simulink model "HSat_orbit_merged_maria"  (R2023b)
settings: Solver=FixedStepAuto  StartTime=0  StopTime=86400*900  MaxStep=3600  RelTol=1e-3  EnableMultiTasking=on
values from neighbouring files (symbols this model uses):
  alpha_acc = sqrt(0.7)    [HSat_op_setup_merged_maria.m]    (also in init_orbit_analysis_with_drag_loss.m)
  ext_ENV_G = 6.674e-11    [HSat_op_setup.m]    (also in HSat_op_setup_merged_maria.m)
  ext_ENV_muEarth = 3.986005e14    (= 398600500000000)    [GEO_insertion_setup.m]    (also in HSat_op_setup.m; HSat_op_setup_merged_maria.m; init_orbit_analysis_with_drag_loss.m)
  ext_ENV_Re = 6.37813700*10^6    (= 6378137)    [HSat_op_setup.m]    (also in HSat_op_setup_merged_maria.m)
  ext_EOR_atmosphere_end = 1000e3    (= 1000000)    [HSat_op_setup.m]    (also in HSat_op_setup_merged_maria.m)
  ext_EOR_perigeeraise_end = 600e3    (= 600000)    [HSat_op_setup.m]    (also in HSat_op_setup_merged_maria.m)
  ext_Main_initDate_IC_T = sim_start    [HSat_op_setup.m]    (also in HSat_op_setup_merged_maria.m)
  ext_SC_activecorr_COE_ECI = [1, 1, 1, 0, 0, 0, 0, 0 ]    [HSat_op_setup.m]    (also in HSat_op_setup_merged_maria.m)
  ext_SC_balanced_COE_ECI = [ .500    0.70    1.100 1 1]    [HSat_op_setup.m]    (also in HSat_op_setup_merged_maria.m = [ 0.10 2.10 1.40    1.0000    1.0000]; launch_settings.m)
  ext_SC_cutofferror_COE_ECI = [150e3, .01, 0.1*pi/180, .1*pi/180,.1*pi/180, 0, 0, 0]    [HSat_op_setup.m]    (also in HSat_op_setup_merged_maria.m)
  ext_SC_init_COE_ECI = [a0,ecc0,i0,an0,ap0,tran0,eccan0,ma0]    [HSat_op_setup.m]    (also in HSat_op_setup_merged_maria.m)
  ext_SC_target_COE_ECI = [a1,ecc1,i1,an1,ap1,tran1,eccan1,ma1]    [HSat_op_setup.m]    (also in HSat_op_setup_merged_maria.m)
  ext_SC_target_lambda = 67*pi/180    (= 1.16937059884)    [HSat_op_setup.m]    (also in HSat_op_setup_merged_maria.m)
  flip_timer = 2*60*60    (= 7200)    [HSat_op_setup_merged_maria.m]
  P_solar = 4.56e-6    (= 4.56e-06)    [HSat_op_setup_merged_maria.m]    (also in init_orbit_analysis_with_drag_loss.m)
  sim_SC_init_CoG_EOR_dry = [-0.00448 0.00106 0.46931]    [HSat_op_setup.m]    (also in HSat_op_setup_merged_maria.m)
  sim_SC_init_CoG_propellant = [0 0 0.24758]    [HSat_op_setup.m]    (also in HSat_op_setup_merged_maria.m)
  sim_SC_init_dry_mass = sim_SC_init_wet_mass-sim_SC_init_propellant_mass    (= 727)    [HSat_op_setup.m]    (also in HSat_op_setup_merged_maria.m = 813.7)
  sim_SC_init_MoI_EOR_wet = [ ... (first row only)    [HSat_op_setup.m]    (also in HSat_op_setup_merged_maria.m; init_orbit_analysis_with_drag_loss.m)
  sim_SC_init_wet_mass = 750    [HSat_op_setup.m]    (also in HSat_op_setup_merged_maria.m)
  sim_thrust_force = [ ... (first row only)    [HSat_op_setup.m]    (also in HSat_op_setup_merged_maria.m)
  sim_thrust_massflow = [ ... (first row only)    [HSat_op_setup.m]    (also in HSat_op_setup_merged_maria.m)
  sim_thrust_vector = [ ... (first row only)    [HSat_op_setup.m]    (also in HSat_op_setup_merged_maria.m)
  sim_thruster_position = [ ... (first row only)    [HSat_op_setup.m]    (also in HSat_op_setup_merged_maria.m)
  sim_ts_save = 60    [HSat_op_setup.m]    (also in HSat_op_setup_merged_maria.m)
  sun_pointing_SA = 0    [HSat_op_setup_merged_maria.m]    (also in init_orbit_analysis_with_drag_loss.m)
  third_body_jupiter = 1    [HSat_op_setup.m]    (also in HSat_op_setup_merged_maria.m)
  third_body_moon = 1    [HSat_op_setup.m]    (also in HSat_op_setup_merged_maria.m)
  third_body_sun = 1    [HSat_op_setup.m]    (also in HSat_op_setup_merged_maria.m)
libraries: aerolibutil x59, simulink x18, matrix_library x16, Toolbox x10, sharedtransform x9, sharedutil x5, aerolibatmos2 x1, simulink_extras x1
(part 7 of 8)

== system HSat_orbit_merged_maria/Subsystem1/control/EORattitude/Subsystem4/Attitude for OR thrusters/q_scb_calc/Yscb x Zscb ==
  a(1) a(2) a(3) : Inport
  b(1) b(2) b(3) : Inport  Port=2
  Product : Product  InputSameDT=on  SaturateOnIntegerOverflow=on  OutDataTypeStr=Inherit: Same as first input
  Product1 : Product  InputSameDT=on  SaturateOnIntegerOverflow=on  OutDataTypeStr=Inherit: Same as first input
  Selector : Selector  InputPortWidth=3  IndexOptions=Index vector (dialog)  Indices=[2 3 1]  OutputSizes=1
  Selector1 : Selector  InputPortWidth=3  IndexOptions=Index vector (dialog)  Indices=[3 1 2]  OutputSizes=1
  Selector2 : Selector  InputPortWidth=3  IndexOptions=Index vector (dialog)  Indices=[2 3 1]  OutputSizes=1
  Selector3 : Selector  InputPortWidth=3  IndexOptions=Index vector (dialog)  Indices=[3 1 2]  OutputSizes=1
  Sum : Sum  Inputs=+|-  InputSameDT=on  SaturateOnIntegerOverflow=on  OutDataTypeStr=Inherit: Same as first input
  c(1) c(2) c(3) : Outport  InitialOutput=0
  wires:
  Sum/1 -> c(1) c(2) c(3)/1
  b(1) b(2) b(3)/1 -> Selector1/1, Selector2/1
  Selector/1 -> Product/1
  a(1) a(2) a(3)/1 -> Selector/1, Selector3/1
  Product/1 -> Sum/1
  Selector1/1 -> Product/2
  Product1/1 -> Sum/2
  Selector2/1 -> Product1/2
  Selector3/1 -> Product1/1

== system HSat_orbit_merged_maria/Subsystem1/control/EORattitude/Subsystem4/Attitude for OR thrusters/q_scb_calc/Zeci x Reci ==
  a(1) a(2) a(3) : Inport
  b(1) b(2) b(3) : Inport  Port=2
  Product : Product  InputSameDT=on  SaturateOnIntegerOverflow=on  OutDataTypeStr=Inherit: Same as first input
  Product1 : Product  InputSameDT=on  SaturateOnIntegerOverflow=on  OutDataTypeStr=Inherit: Same as first input
  Selector : Selector  InputPortWidth=3  IndexOptions=Index vector (dialog)  Indices=[2 3 1]  OutputSizes=1
  Selector1 : Selector  InputPortWidth=3  IndexOptions=Index vector (dialog)  Indices=[3 1 2]  OutputSizes=1
  Selector2 : Selector  InputPortWidth=3  IndexOptions=Index vector (dialog)  Indices=[2 3 1]  OutputSizes=1
  Selector3 : Selector  InputPortWidth=3  IndexOptions=Index vector (dialog)  Indices=[3 1 2]  OutputSizes=1
  Sum : Sum  Inputs=+|-  InputSameDT=on  SaturateOnIntegerOverflow=on  OutDataTypeStr=Inherit: Same as first input
  c(1) c(2) c(3) : Outport  InitialOutput=0
  wires:
  Selector3/1 -> Product1/1
  Selector2/1 -> Product1/2
  Product1/1 -> Sum/2
  Selector1/1 -> Product/2
  Product/1 -> Sum/1
  a(1) a(2) a(3)/1 -> Selector3/1, Selector/1
  Selector/1 -> Product/1
  b(1) b(2) b(3)/1 -> Selector2/1, Selector1/1
  Sum/1 -> c(1) c(2) c(3)/1

== system HSat_orbit_merged_maria/Subsystem1/control/EORattitude/Subsystem4/Attitude for SK unloading/Subsystem/VecNormalize4 ==
  In1 : Inport
  Constant : Constant
  Demux : Demux  Outputs=[-1 1]
  Divide : Product  Inputs=*/  OutDataTypeStr=double
  Ground : Ground
  Math Function : Math  Operator=square  SignedPower=on
  Math Function1 : Math  Operator=sqrt  SignedPower=on
  Mux : Mux  Inputs=2
  Mux1 : Mux  Inputs=2
  Product : Product  RndMeth=Zero
  Sum of Elements : Sum  Inputs=+
  Switch : Switch  Criteria=u2 > Threshold  Threshold=eps  SaturateOnIntegerOverflow=off  InputSameDT=off
  Out1 : Outport  VectorParamsAs1DForOutWhenUnconnected=off
  wires:
  Math Function/1 -> Sum of Elements/1
  Demux/1 -> Divide/1
  Constant/1 -> Mux1/2
  Mux1/1 -> Switch/3
  Divide/1 -> Out1/1
  Switch/1 -> Demux/1
  Mux/1 -> Switch/1
  Demux/2 -> Divide/2
  Product/1 -> Mux1/1
  In1/1 -> Product/1, Math Function/1, Mux/1
  Ground/1 -> Product/2
  Sum of Elements/1 -> Math Function1/1
  Math Function1/1 -> Mux/2, Switch/2

== system HSat_orbit_merged_maria/Subsystem1/control/EORattitude/Subsystem4/Attitude for SK unloading/Subsystem/Zeci x Reci ==
  a(1) a(2) a(3) : Inport
  b(1) b(2) b(3) : Inport  Port=2
  Product : Product  InputSameDT=on  SaturateOnIntegerOverflow=on  OutDataTypeStr=Inherit: Same as first input
  Product1 : Product  InputSameDT=on  SaturateOnIntegerOverflow=on  OutDataTypeStr=Inherit: Same as first input
  Selector : Selector  InputPortWidth=3  IndexOptions=Index vector (dialog)  Indices=[2 3 1]  OutputSizes=1
  Selector1 : Selector  InputPortWidth=3  IndexOptions=Index vector (dialog)  Indices=[3 1 2]  OutputSizes=1
  Selector2 : Selector  InputPortWidth=3  IndexOptions=Index vector (dialog)  Indices=[2 3 1]  OutputSizes=1
  Selector3 : Selector  InputPortWidth=3  IndexOptions=Index vector (dialog)  Indices=[3 1 2]  OutputSizes=1
  Sum : Sum  Inputs=+|-  InputSameDT=on  SaturateOnIntegerOverflow=on  OutDataTypeStr=Inherit: Same as first input
  c(1) c(2) c(3) : Outport  InitialOutput=0
  wires:
  Selector3/1 -> Product1/1
  Selector2/1 -> Product1/2
  Product1/1 -> Sum/2
  Selector1/1 -> Product/2
  Product/1 -> Sum/1
  a(1) a(2) a(3)/1 -> Selector3/1, Selector/1
  Selector/1 -> Product/1
  b(1) b(2) b(3)/1 -> Selector2/1, Selector1/1
  Sum/1 -> c(1) c(2) c(3)/1

== system HSat_orbit_merged_maria/Subsystem1/control/EORattitude/Subsystem4/Attitude for SK unloading/Subsystem/Zeci x Reci1 ==
  a(1) a(2) a(3) : Inport
  b(1) b(2) b(3) : Inport  Port=2
  Product : Product  InputSameDT=on  SaturateOnIntegerOverflow=on  OutDataTypeStr=Inherit: Same as first input
  Product1 : Product  InputSameDT=on  SaturateOnIntegerOverflow=on  OutDataTypeStr=Inherit: Same as first input
  Selector : Selector  InputPortWidth=3  IndexOptions=Index vector (dialog)  Indices=[2 3 1]  OutputSizes=1
  Selector1 : Selector  InputPortWidth=3  IndexOptions=Index vector (dialog)  Indices=[3 1 2]  OutputSizes=1
  Selector2 : Selector  InputPortWidth=3  IndexOptions=Index vector (dialog)  Indices=[2 3 1]  OutputSizes=1
  Selector3 : Selector  InputPortWidth=3  IndexOptions=Index vector (dialog)  Indices=[3 1 2]  OutputSizes=1
  Sum : Sum  Inputs=+|-  InputSameDT=on  SaturateOnIntegerOverflow=on  OutDataTypeStr=Inherit: Same as first input
  c(1) c(2) c(3) : Outport  InitialOutput=0
  wires:
  Selector3/1 -> Product1/1
  Selector2/1 -> Product1/2
  Product1/1 -> Sum/2
  Selector1/1 -> Product/2
  Product/1 -> Sum/1
  a(1) a(2) a(3)/1 -> Selector3/1, Selector/1
  Selector/1 -> Product/1
  b(1) b(2) b(3)/1 -> Selector2/1, Selector1/1
  Sum/1 -> c(1) c(2) c(3)/1

== system HSat_orbit_merged_maria/Subsystem1/control/EORattitude/Subsystem4/Subsystem3/FlipSatellite/VecNormalize ==
  In1 : Inport
  Constant : Constant
  Demux : Demux  Outputs=[-1 1]
  Divide : Product  Inputs=*/  OutDataTypeStr=double
  Ground : Ground
  Math Function : Math  Operator=square  SignedPower=on
  Math Function1 : Math  Operator=sqrt  SignedPower=on
  Mux : Mux  Inputs=2
  Mux1 : Mux  Inputs=2
  Product : Product  RndMeth=Zero
  Sum of Elements : Sum  Inputs=+
  Switch : Switch  Criteria=u2 > Threshold  Threshold=eps  SaturateOnIntegerOverflow=off  InputSameDT=off
  Out1 : Outport  VectorParamsAs1DForOutWhenUnconnected=off
  wires:
  Math Function/1 -> Sum of Elements/1
  Demux/1 -> Divide/1
  Constant/1 -> Mux1/2
  Mux1/1 -> Switch/3
  Divide/1 -> Out1/1
  Switch/1 -> Demux/1
  Mux/1 -> Switch/1
  Demux/2 -> Divide/2
  Product/1 -> Mux1/1
  In1/1 -> Product/1, Math Function/1, Mux/1
  Ground/1 -> Product/2
  Sum of Elements/1 -> Math Function1/1
  Math Function1/1 -> Mux/2, Switch/2

== system HSat_orbit_merged_maria/Subsystem1/control/EORattitude/Subsystem4/Subsystem3/FlipSatellite/VecNormalize1 ==
  In1 : Inport
  Constant : Constant
  Demux : Demux  Outputs=[-1 1]
  Divide : Product  Inputs=*/  OutDataTypeStr=double
  Ground : Ground
  Math Function : Math  Operator=square  SignedPower=on
  Math Function1 : Math  Operator=sqrt  SignedPower=on
  Mux : Mux  Inputs=2
  Mux1 : Mux  Inputs=2
  Product : Product  RndMeth=Zero
  Sum of Elements : Sum  Inputs=+
  Switch : Switch  Criteria=u2 > Threshold  Threshold=eps  SaturateOnIntegerOverflow=off  InputSameDT=off
  Out1 : Outport  VectorParamsAs1DForOutWhenUnconnected=off
  wires:
  Math Function/1 -> Sum of Elements/1
  Demux/1 -> Divide/1
  Constant/1 -> Mux1/2
  Mux1/1 -> Switch/3
  Divide/1 -> Out1/1
  Switch/1 -> Demux/1
  Mux/1 -> Switch/1
  Demux/2 -> Divide/2
  Product/1 -> Mux1/1
  In1/1 -> Product/1, Math Function/1, Mux/1
  Ground/1 -> Product/2
  Sum of Elements/1 -> Math Function1/1
  Math Function1/1 -> Mux/2, Switch/2

== system HSat_orbit_merged_maria/Subsystem1/control/Subsystem6/Subsystem2/Subsystem1/Subsystem/VecNormalize4 ==
  In1 : Inport
  Constant : Constant
  Demux : Demux  Outputs=[-1 1]
  Divide : Product  Inputs=*/  OutDataTypeStr=double
  Ground : Ground
  Math Function : Math  Operator=square  SignedPower=on
  Math Function1 : Math  Operator=sqrt  SignedPower=on
  Mux : Mux  Inputs=2
  Mux1 : Mux  Inputs=2
  Product : Product  RndMeth=Zero
  Sum of Elements : Sum  Inputs=+
  Switch : Switch  Criteria=u2 > Threshold  Threshold=eps  SaturateOnIntegerOverflow=off  InputSameDT=off
  Out1 : Outport  VectorParamsAs1DForOutWhenUnconnected=off
  wires:
  Math Function/1 -> Sum of Elements/1
  Demux/1 -> Divide/1
  Constant/1 -> Mux1/2
  Mux1/1 -> Switch/3
  Divide/1 -> Out1/1
  Switch/1 -> Demux/1
  Mux/1 -> Switch/1
  Demux/2 -> Divide/2
  Product/1 -> Mux1/1
  In1/1 -> Product/1, Math Function/1, Mux/1
  Ground/1 -> Product/2
  Sum of Elements/1 -> Math Function1/1
  Math Function1/1 -> Mux/2, Switch/2

== system HSat_orbit_merged_maria/Subsystem1/control/Subsystem6/Subsystem2/Subsystem1/Subsystem/Zeci x Reci ==
  a(1) a(2) a(3) : Inport
  b(1) b(2) b(3) : Inport  Port=2
  Product : Product  InputSameDT=on  SaturateOnIntegerOverflow=on  OutDataTypeStr=Inherit: Same as first input
  Product1 : Product  InputSameDT=on  SaturateOnIntegerOverflow=on  OutDataTypeStr=Inherit: Same as first input
  Selector : Selector  InputPortWidth=3  IndexOptions=Index vector (dialog)  Indices=[2 3 1]  OutputSizes=1
  Selector1 : Selector  InputPortWidth=3  IndexOptions=Index vector (dialog)  Indices=[3 1 2]  OutputSizes=1
  Selector2 : Selector  InputPortWidth=3  IndexOptions=Index vector (dialog)  Indices=[2 3 1]  OutputSizes=1
  Selector3 : Selector  InputPortWidth=3  IndexOptions=Index vector (dialog)  Indices=[3 1 2]  OutputSizes=1
  Sum : Sum  Inputs=+|-  InputSameDT=on  SaturateOnIntegerOverflow=on  OutDataTypeStr=Inherit: Same as first input
  c(1) c(2) c(3) : Outport  InitialOutput=0
  wires:
  Selector3/1 -> Product1/1
  Selector2/1 -> Product1/2
  Product1/1 -> Sum/2
  Selector1/1 -> Product/2
  Product/1 -> Sum/1
  a(1) a(2) a(3)/1 -> Selector3/1, Selector/1
  Selector/1 -> Product/1
  b(1) b(2) b(3)/1 -> Selector2/1, Selector1/1
  Sum/1 -> c(1) c(2) c(3)/1

== system HSat_orbit_merged_maria/Subsystem1/control/Subsystem6/Subsystem2/Subsystem1/Subsystem/Zeci x Reci1 ==
  a(1) a(2) a(3) : Inport
  b(1) b(2) b(3) : Inport  Port=2
  Product : Product  InputSameDT=on  SaturateOnIntegerOverflow=on  OutDataTypeStr=Inherit: Same as first input
  Product1 : Product  InputSameDT=on  SaturateOnIntegerOverflow=on  OutDataTypeStr=Inherit: Same as first input
  Selector : Selector  InputPortWidth=3  IndexOptions=Index vector (dialog)  Indices=[2 3 1]  OutputSizes=1
  Selector1 : Selector  InputPortWidth=3  IndexOptions=Index vector (dialog)  Indices=[3 1 2]  OutputSizes=1
  Selector2 : Selector  InputPortWidth=3  IndexOptions=Index vector (dialog)  Indices=[2 3 1]  OutputSizes=1
  Selector3 : Selector  InputPortWidth=3  IndexOptions=Index vector (dialog)  Indices=[3 1 2]  OutputSizes=1
  Sum : Sum  Inputs=+|-  InputSameDT=on  SaturateOnIntegerOverflow=on  OutDataTypeStr=Inherit: Same as first input
  c(1) c(2) c(3) : Outport  InitialOutput=0
  wires:
  Selector3/1 -> Product1/1
  Selector2/1 -> Product1/2
  Product1/1 -> Sum/2
  Selector1/1 -> Product/2
  Product/1 -> Sum/1
  a(1) a(2) a(3)/1 -> Selector3/1, Selector/1
  Selector/1 -> Product/1
  b(1) b(2) b(3)/1 -> Selector2/1, Selector1/1
  Sum/1 -> c(1) c(2) c(3)/1

== system HSat_orbit_merged_maria/Subsystem1/control/Subsystem6/Subsystem2/Subsystem1/q_scb_calc/VecNormalize ==
  In1 : Inport
  Constant : Constant
  Demux : Demux  Outputs=[-1 1]
  Divide : Product  Inputs=*/  OutDataTypeStr=double
  Ground : Ground
  Math Function : Math  Operator=square  SignedPower=on
  Math Function1 : Math  Operator=sqrt  SignedPower=on
  Mux : Mux  Inputs=2
  Mux1 : Mux  Inputs=2
  Product : Product  RndMeth=Zero
  Sum of Elements : Sum  Inputs=+
  Switch : Switch  Criteria=u2 > Threshold  Threshold=eps  SaturateOnIntegerOverflow=off  InputSameDT=off
  Out1 : Outport  VectorParamsAs1DForOutWhenUnconnected=off
  wires:
  Math Function/1 -> Sum of Elements/1
  Demux/1 -> Divide/1
  Constant/1 -> Mux1/2
  Mux1/1 -> Switch/3
  Divide/1 -> Out1/1
  Switch/1 -> Demux/1
  Mux/1 -> Switch/1
  Demux/2 -> Divide/2
  Product/1 -> Mux1/1
  In1/1 -> Product/1, Math Function/1, Mux/1
  Ground/1 -> Product/2
  Sum of Elements/1 -> Math Function1/1
  Math Function1/1 -> Mux/2, Switch/2

== system HSat_orbit_merged_maria/Subsystem1/control/Subsystem6/Subsystem2/Subsystem1/q_scb_calc/VecNormalize1 ==
  In1 : Inport
  Constant : Constant
  Demux : Demux  Outputs=[-1 1]
  Divide : Product  Inputs=*/  OutDataTypeStr=double
  Ground : Ground
  Math Function : Math  Operator=square  SignedPower=on
  Math Function1 : Math  Operator=sqrt  SignedPower=on
  Mux : Mux  Inputs=2
  Mux1 : Mux  Inputs=2
  Product : Product  RndMeth=Zero
  Sum of Elements : Sum  Inputs=+
  Switch : Switch  Criteria=u2 > Threshold  Threshold=eps  SaturateOnIntegerOverflow=off  InputSameDT=off
  Out1 : Outport  VectorParamsAs1DForOutWhenUnconnected=off
  wires:
  Math Function/1 -> Sum of Elements/1
  Demux/1 -> Divide/1
  Constant/1 -> Mux1/2
  Mux1/1 -> Switch/3
  Divide/1 -> Out1/1
  Switch/1 -> Demux/1
  Mux/1 -> Switch/1
  Demux/2 -> Divide/2
  Product/1 -> Mux1/1
  In1/1 -> Product/1, Math Function/1, Mux/1
  Ground/1 -> Product/2
  Sum of Elements/1 -> Math Function1/1
  Math Function1/1 -> Mux/2, Switch/2

== system HSat_orbit_merged_maria/Subsystem1/control/Subsystem6/Subsystem2/Subsystem1/q_scb_calc/VecNormalize2 ==
  In1 : Inport
  Constant : Constant
  Demux : Demux  Outputs=[-1 1]
  Divide : Product  Inputs=*/  OutDataTypeStr=double
  Ground : Ground
  Math Function : Math  Operator=square  SignedPower=on
  Math Function1 : Math  Operator=sqrt  SignedPower=on
  Mux : Mux  Inputs=2
  Mux1 : Mux  Inputs=2
  Product : Product  RndMeth=Zero
  Sum of Elements : Sum  Inputs=+
  Switch : Switch  Criteria=u2 > Threshold  Threshold=eps  SaturateOnIntegerOverflow=off  InputSameDT=off
  Out1 : Outport  VectorParamsAs1DForOutWhenUnconnected=off
  wires:
  Math Function/1 -> Sum of Elements/1
  Demux/1 -> Divide/1
  Constant/1 -> Mux1/2
  Mux1/1 -> Switch/3
  Divide/1 -> Out1/1
  Switch/1 -> Demux/1
  Mux/1 -> Switch/1
  Demux/2 -> Divide/2
  Product/1 -> Mux1/1
  In1/1 -> Product/1, Math Function/1, Mux/1
  Ground/1 -> Product/2
  Sum of Elements/1 -> Math Function1/1
  Math Function1/1 -> Mux/2, Switch/2

== system HSat_orbit_merged_maria/Subsystem1/control/Subsystem6/Subsystem2/Subsystem1/q_scb_calc/VecNormalize3 ==
  In1 : Inport
  Constant : Constant
  Demux : Demux  Outputs=[-1 1]
  Divide : Product  Inputs=*/  OutDataTypeStr=double
  Ground : Ground
  Math Function : Math  Operator=square  SignedPower=on
  Math Function1 : Math  Operator=sqrt  SignedPower=on
  Mux : Mux  Inputs=2
  Mux1 : Mux  Inputs=2
  Product : Product  RndMeth=Zero
  Sum of Elements : Sum  Inputs=+
  Switch : Switch  Criteria=u2 > Threshold  Threshold=eps  SaturateOnIntegerOverflow=off  InputSameDT=off
  Out1 : Outport  VectorParamsAs1DForOutWhenUnconnected=off
  wires:
  Math Function/1 -> Sum of Elements/1
  Demux/1 -> Divide/1
  Constant/1 -> Mux1/2
  Mux1/1 -> Switch/3
  Divide/1 -> Out1/1
  Switch/1 -> Demux/1
  Mux/1 -> Switch/1
  Demux/2 -> Divide/2
  Product/1 -> Mux1/1
  In1/1 -> Product/1, Math Function/1, Mux/1
  Ground/1 -> Product/2
  Sum of Elements/1 -> Math Function1/1
  Math Function1/1 -> Mux/2, Switch/2

== system HSat_orbit_merged_maria/Subsystem1/control/Subsystem6/Subsystem2/Subsystem1/q_scb_calc/Yscb x Zscb ==
  a(1) a(2) a(3) : Inport
  b(1) b(2) b(3) : Inport  Port=2
  Product : Product  InputSameDT=on  SaturateOnIntegerOverflow=on  OutDataTypeStr=Inherit: Same as first input
  Product1 : Product  InputSameDT=on  SaturateOnIntegerOverflow=on  OutDataTypeStr=Inherit: Same as first input
  Selector : Selector  InputPortWidth=3  IndexOptions=Index vector (dialog)  Indices=[2 3 1]  OutputSizes=1
  Selector1 : Selector  InputPortWidth=3  IndexOptions=Index vector (dialog)  Indices=[3 1 2]  OutputSizes=1
  Selector2 : Selector  InputPortWidth=3  IndexOptions=Index vector (dialog)  Indices=[2 3 1]  OutputSizes=1
  Selector3 : Selector  InputPortWidth=3  IndexOptions=Index vector (dialog)  Indices=[3 1 2]  OutputSizes=1
  Sum : Sum  Inputs=+|-  InputSameDT=on  SaturateOnIntegerOverflow=on  OutDataTypeStr=Inherit: Same as first input
  c(1) c(2) c(3) : Outport  InitialOutput=0
  wires:
  Sum/1 -> c(1) c(2) c(3)/1
  b(1) b(2) b(3)/1 -> Selector1/1, Selector2/1
  Selector/1 -> Product/1
  a(1) a(2) a(3)/1 -> Selector/1, Selector3/1
  Product/1 -> Sum/1
  Selector1/1 -> Product/2
  Product1/1 -> Sum/2
  Selector2/1 -> Product1/2
  Selector3/1 -> Product1/1

== system HSat_orbit_merged_maria/Subsystem1/control/Subsystem6/Subsystem2/Subsystem1/q_scb_calc/Zeci x Reci ==
  a(1) a(2) a(3) : Inport
  b(1) b(2) b(3) : Inport  Port=2
  Product : Product  InputSameDT=on  SaturateOnIntegerOverflow=on  OutDataTypeStr=Inherit: Same as first input
  Product1 : Product  InputSameDT=on  SaturateOnIntegerOverflow=on  OutDataTypeStr=Inherit: Same as first input
  Selector : Selector  InputPortWidth=3  IndexOptions=Index vector (dialog)  Indices=[2 3 1]  OutputSizes=1
  Selector1 : Selector  InputPortWidth=3  IndexOptions=Index vector (dialog)  Indices=[3 1 2]  OutputSizes=1
  Selector2 : Selector  InputPortWidth=3  IndexOptions=Index vector (dialog)  Indices=[2 3 1]  OutputSizes=1
  Selector3 : Selector  InputPortWidth=3  IndexOptions=Index vector (dialog)  Indices=[3 1 2]  OutputSizes=1
  Sum : Sum  Inputs=+|-  InputSameDT=on  SaturateOnIntegerOverflow=on  OutDataTypeStr=Inherit: Same as first input
  c(1) c(2) c(3) : Outport  InitialOutput=0
  wires:
  Selector3/1 -> Product1/1
  Selector2/1 -> Product1/2
  Product1/1 -> Sum/2
  Selector1/1 -> Product/2
  Product/1 -> Sum/1
  a(1) a(2) a(3)/1 -> Selector3/1, Selector/1
  Selector/1 -> Product/1
  b(1) b(2) b(3)/1 -> Selector2/1, Selector1/1
  Sum/1 -> c(1) c(2) c(3)/1

== system HSat_orbit_merged_maria/Subsystem1/Dynamics/disturbing torques/Disturbing torques/sc area projected to v // aero drag torque // srp torque/Switch Case Action Subsystem/sun pointing solar arrays/Nomalize_noDivideByZero1 ==
  e : Inport
  2-norm : Subsystem
      mask Display: disp('||u||')
  Product : Product  Inputs=*/  InputSameDT=on  RndMeth=Zero  SaturateOnIntegerOverflow=on  OutDataTypeStr=Inherit: Same as first input
  Switch : Switch  Criteria=u2 > Threshold  SaturateOnIntegerOverflow=off  InputSameDT=off
  zero : Constant  Value=0
  ehat : Outport
  wires:
  e/1 -> 2-norm/1(In1), Product/1
  2-norm/1(Out1) -> Switch/2, Product/2
  Switch/1 -> ehat/1
  Product/1 -> Switch/1
  zero/1 -> Switch/3

== system HSat_orbit_merged_maria/Subsystem1/Dynamics/disturbing torques/Disturbing torques/sc area projected to v // aero drag torque // srp torque/z -1/Nomalize_noDivideByZero/2-norm ==
  In1 : Inport
  Math Function : Math  Operator=sqrt  SignedPower=on
  Product1 : Product  InputSameDT=on  RndMeth=Zero  SaturateOnIntegerOverflow=on  OutDataTypeStr=Inherit: Same as first input
  Sum : Sum  Inputs=+  InputSameDT=on  SaturateOnIntegerOverflow=on  OutDataTypeStr=Inherit: Same as first input
  Out1 : Outport
  wires:
  In1/1 -> Product1/1, Product1/2
  Product1/1 -> Sum/1
  Sum/1 -> Math Function/1
  Math Function/1 -> Out1/1

== system HSat_orbit_merged_maria/Subsystem1/Dynamics/disturbing torques/Disturbing torques/sc area projected to v // aero drag torque // srp torque/z -1/Nomalize_noDivideByZero1/2-norm ==
  In1 : Inport
  Math Function : Math  Operator=sqrt  SignedPower=on
  Product1 : Product  InputSameDT=on  RndMeth=Zero  SaturateOnIntegerOverflow=on  OutDataTypeStr=Inherit: Same as first input
  Sum : Sum  Inputs=+  InputSameDT=on  SaturateOnIntegerOverflow=on  OutDataTypeStr=Inherit: Same as first input
  Out1 : Outport
  wires:
  In1/1 -> Product1/1, Product1/2
  Product1/1 -> Sum/1
  Sum/1 -> Math Function/1
  Math Function/1 -> Out1/1

== system HSat_orbit_merged_maria/Subsystem1/Dynamics/disturbing torques/Disturbing torques/sc area projected to v // aero drag torque // srp torque/z -2/Nomalize_noDivideByZero/2-norm ==
  In1 : Inport
  Math Function : Math  Operator=sqrt  SignedPower=on
  Product1 : Product  InputSameDT=on  RndMeth=Zero  SaturateOnIntegerOverflow=on  OutDataTypeStr=Inherit: Same as first input
  Sum : Sum  Inputs=+  InputSameDT=on  SaturateOnIntegerOverflow=on  OutDataTypeStr=Inherit: Same as first input
  Out1 : Outport
  wires:
  In1/1 -> Product1/1, Product1/2
  Product1/1 -> Sum/1
  Sum/1 -> Math Function/1
  Math Function/1 -> Out1/1

== system HSat_orbit_merged_maria/Subsystem1/Dynamics/disturbing torques/Disturbing torques/sc area projected to v // aero drag torque // srp torque/z -2/Nomalize_noDivideByZero1/2-norm ==
  In1 : Inport
  Math Function : Math  Operator=sqrt  SignedPower=on
  Product1 : Product  InputSameDT=on  RndMeth=Zero  SaturateOnIntegerOverflow=on  OutDataTypeStr=Inherit: Same as first input
  Sum : Sum  Inputs=+  InputSameDT=on  SaturateOnIntegerOverflow=on  OutDataTypeStr=Inherit: Same as first input
  Out1 : Outport
  wires:
  In1/1 -> Product1/1, Product1/2
  Product1/1 -> Sum/1
  Sum/1 -> Math Function/1
  Math Function/1 -> Out1/1

== system HSat_orbit_merged_maria/Subsystem1/Dynamics/disturbing torques/Disturbing torques/sc area projected to v // aero drag torque // srp torque/z -3/Nomalize_noDivideByZero/2-norm ==
  In1 : Inport
  Math Function : Math  Operator=sqrt  SignedPower=on
  Product1 : Product  InputSameDT=on  RndMeth=Zero  SaturateOnIntegerOverflow=on  OutDataTypeStr=Inherit: Same as first input
  Sum : Sum  Inputs=+  InputSameDT=on  SaturateOnIntegerOverflow=on  OutDataTypeStr=Inherit: Same as first input
  Out1 : Outport
  wires:
  In1/1 -> Product1/1, Product1/2
  Product1/1 -> Sum/1
  Sum/1 -> Math Function/1
  Math Function/1 -> Out1/1

== system HSat_orbit_merged_maria/Subsystem1/Dynamics/disturbing torques/Disturbing torques/sc area projected to v // aero drag torque // srp torque/z -3/Nomalize_noDivideByZero1/2-norm ==
  In1 : Inport
  Math Function : Math  Operator=sqrt  SignedPower=on
  Product1 : Product  InputSameDT=on  RndMeth=Zero  SaturateOnIntegerOverflow=on  OutDataTypeStr=Inherit: Same as first input
  Sum : Sum  Inputs=+  InputSameDT=on  SaturateOnIntegerOverflow=on  OutDataTypeStr=Inherit: Same as first input
  Out1 : Outport
  wires:
  In1/1 -> Product1/1, Product1/2
  Product1/1 -> Sum/1
  Sum/1 -> Math Function/1
  Math Function/1 -> Out1/1

== system HSat_orbit_merged_maria/Subsystem1/Dynamics/disturbing torques/Disturbing torques/sc area projected to v // aero drag torque // srp torque/z -4/Nomalize_noDivideByZero/2-norm ==
  In1 : Inport
  Math Function : Math  Operator=sqrt  SignedPower=on
  Product1 : Product  InputSameDT=on  RndMeth=Zero  SaturateOnIntegerOverflow=on  OutDataTypeStr=Inherit: Same as first input
  Sum : Sum  Inputs=+  InputSameDT=on  SaturateOnIntegerOverflow=on  OutDataTypeStr=Inherit: Same as first input
  Out1 : Outport
  wires:
  In1/1 -> Product1/1, Product1/2
  Product1/1 -> Sum/1
  Sum/1 -> Math Function/1
  Math Function/1 -> Out1/1

== system HSat_orbit_merged_maria/Subsystem1/Dynamics/disturbing torques/Disturbing torques/sc area projected to v // aero drag torque // srp torque/z -4/Nomalize_noDivideByZero1/2-norm ==
  In1 : Inport
  Math Function : Math  Operator=sqrt  SignedPower=on
  Product1 : Product  InputSameDT=on  RndMeth=Zero  SaturateOnIntegerOverflow=on  OutDataTypeStr=Inherit: Same as first input
  Sum : Sum  Inputs=+  InputSameDT=on  SaturateOnIntegerOverflow=on  OutDataTypeStr=Inherit: Same as first input
  Out1 : Outport
  wires:
  In1/1 -> Product1/1, Product1/2
  Product1/1 -> Sum/1
  Sum/1 -> Math Function/1
  Math Function/1 -> Out1/1

== system HSat_orbit_merged_maria/Subsystem1/Dynamics/disturbing torques/Disturbing torques/sc area projected to v // aero drag torque // srp torque/z -5/Nomalize_noDivideByZero/2-norm ==
  In1 : Inport
  Math Function : Math  Operator=sqrt  SignedPower=on
  Product1 : Product  InputSameDT=on  RndMeth=Zero  SaturateOnIntegerOverflow=on  OutDataTypeStr=Inherit: Same as first input
  Sum : Sum  Inputs=+  InputSameDT=on  SaturateOnIntegerOverflow=on  OutDataTypeStr=Inherit: Same as first input
  Out1 : Outport
  wires:
  In1/1 -> Product1/1, Product1/2
  Product1/1 -> Sum/1
  Sum/1 -> Math Function/1
  Math Function/1 -> Out1/1

== system HSat_orbit_merged_maria/Subsystem1/Dynamics/disturbing torques/Disturbing torques/sc area projected to v // aero drag torque // srp torque/z -5/Nomalize_noDivideByZero1/2-norm ==
  In1 : Inport
  Math Function : Math  Operator=sqrt  SignedPower=on
  Product1 : Product  InputSameDT=on  RndMeth=Zero  SaturateOnIntegerOverflow=on  OutDataTypeStr=Inherit: Same as first input
  Sum : Sum  Inputs=+  InputSameDT=on  SaturateOnIntegerOverflow=on  OutDataTypeStr=Inherit: Same as first input
  Out1 : Outport
  wires:
  In1/1 -> Product1/1, Product1/2
  Product1/1 -> Sum/1
  Sum/1 -> Math Function/1
  Math Function/1 -> Out1/1

== system HSat_orbit_merged_maria/Subsystem1/Dynamics/disturbing torques/Disturbing torques/sc area projected to v // aero drag torque // srp torque/z -6/Nomalize_noDivideByZero/2-norm ==
  In1 : Inport
  Math Function : Math  Operator=sqrt  SignedPower=on
  Product1 : Product  InputSameDT=on  RndMeth=Zero  SaturateOnIntegerOverflow=on  OutDataTypeStr=Inherit: Same as first input
  Sum : Sum  Inputs=+  InputSameDT=on  SaturateOnIntegerOverflow=on  OutDataTypeStr=Inherit: Same as first input
  Out1 : Outport
  wires:
  In1/1 -> Product1/1, Product1/2
  Product1/1 -> Sum/1
  Sum/1 -> Math Function/1
  Math Function/1 -> Out1/1

== system HSat_orbit_merged_maria/Subsystem1/Dynamics/disturbing torques/Disturbing torques/sc area projected to v // aero drag torque // srp torque/z -6/Nomalize_noDivideByZero1/2-norm ==
  In1 : Inport
  Math Function : Math  Operator=sqrt  SignedPower=on
  Product1 : Product  InputSameDT=on  RndMeth=Zero  SaturateOnIntegerOverflow=on  OutDataTypeStr=Inherit: Same as first input
  Sum : Sum  Inputs=+  InputSameDT=on  SaturateOnIntegerOverflow=on  OutDataTypeStr=Inherit: Same as first input
  Out1 : Outport
  wires:
  In1/1 -> Product1/1, Product1/2
  Product1/1 -> Sum/1
  Sum/1 -> Math Function/1
  Math Function/1 -> Out1/1

== system HSat_orbit_merged_maria/Subsystem1/Dynamics/disturbing torques/Disturbing torques/sc area projected to v // aero drag torque // srp torque/z -7/Nomalize_noDivideByZero/2-norm ==
  In1 : Inport
  Math Function : Math  Operator=sqrt  SignedPower=on
  Product1 : Product  InputSameDT=on  RndMeth=Zero  SaturateOnIntegerOverflow=on  OutDataTypeStr=Inherit: Same as first input
  Sum : Sum  Inputs=+  InputSameDT=on  SaturateOnIntegerOverflow=on  OutDataTypeStr=Inherit: Same as first input
  Out1 : Outport
  wires:
  In1/1 -> Product1/1, Product1/2
  Product1/1 -> Sum/1
  Sum/1 -> Math Function/1
  Math Function/1 -> Out1/1

== system HSat_orbit_merged_maria/Subsystem1/Dynamics/disturbing torques/Disturbing torques/sc area projected to v // aero drag torque // srp torque/z -7/Nomalize_noDivideByZero1/2-norm ==
  In1 : Inport
  Math Function : Math  Operator=sqrt  SignedPower=on
  Product1 : Product  InputSameDT=on  RndMeth=Zero  SaturateOnIntegerOverflow=on  OutDataTypeStr=Inherit: Same as first input
  Sum : Sum  Inputs=+  InputSameDT=on  SaturateOnIntegerOverflow=on  OutDataTypeStr=Inherit: Same as first input
  Out1 : Outport
  wires:
  In1/1 -> Product1/1, Product1/2
  Product1/1 -> Sum/1
  Sum/1 -> Math Function/1
  Math Function/1 -> Out1/1

== system HSat_orbit_merged_maria/Subsystem1/Dynamics/disturbing torques/Disturbing torques/sc area projected to v // aero drag torque // srp torque/Switch Case Action Subsystem/sun pointing solar arrays/Nomalize_noDivideByZero1/2-norm ==
  In1 : Inport
  Math Function : Math  Operator=sqrt  SignedPower=on
  Product1 : Product  InputSameDT=on  RndMeth=Zero  SaturateOnIntegerOverflow=on  OutDataTypeStr=Inherit: Same as first input
  Sum : Sum  Inputs=+  InputSameDT=on  SaturateOnIntegerOverflow=on  OutDataTypeStr=Inherit: Same as first input
  Out1 : Outport
  wires:
  In1/1 -> Product1/1, Product1/2
  Product1/1 -> Sum/1
  Sum/1 -> Math Function/1
  Math Function/1 -> Out1/1

== matlab function HSat_orbit_merged_maria/Subsystem1/Guidance/MATLAB Function1 ==
  data: coe input; nT_slo output; coe1 input; coe0 input; cutoff_coe input; activecorr_coe input; eff output; weights output; krondelta output; activecorr_coe output; balanced_coe input
function [nT_slo, eff, weights, krondelta, activecorr_coe]  = thrustAngle(coe,coe1, coe0,cutoff_coe,activecorr_coe,balanced_coe)

%  constmath;
small=1e-10;
infinite  = 999999.9;
undefined = 999999.1;
% -------------------------  mathematical  --------------------
rad    = 180.0 / pi;
twopi  = 2.0 * pi;
halfpi = pi * 0.5;

% constastro;  % don't overwrite mu
mu=3.986005e14;
muin = mu; % this is the km version

sma=coe(1);
ecc=coe(2);
incl=coe(3);
an=coe(4);
ap=coe(5);
tran    =coe(6);
eccan   =coe(7);
ma      =coe(8);
arglat  =coe(9);
truelon =coe(10);
lonper  =coe(11);


if ( ecc < small )
    % ----------------  circular equatorial  ------------------
    if (incl<small) || ( abs(incl-pi)< small )
        ap = 0.0;
        an= 0.0;
        tran   = truelon;
    else
        % --------------  circular inclined  ------------------
        argp= 0.0;
        nu  = arglat;
    end
else
    % ---------------  elliptical equatorial  -----------------
    if ( ( incl<small) || (abs(incl-pi)<small) )
        ap = lonper;
        an= 0.0;
    end
end

rp0=coe0(1)*(1-coe0(2)^2)/(1+coe0(2)*cos(0));

mu=3.986005e14;
V = sqrt(mu/coe(1));
V0 = sqrt(mu/coe0(1));
V1 = sqrt(mu/coe1(1));

r  = coe(1)*(1-coe(2)^2)/(1+coe(6));
r0  = coe0(1)*(1-coe0(2)^2)/(1+coe0(6));
r1  = coe1(1)*(1-coe1(2)^2)/(1+coe1(6));

v  = sqrt(mu*(2/r-1/coe(1)));
v0 = sqrt(mu*(2/r0-1/coe0(1)));
v1 = sqrt(mu*(2/r1-1/coe1(1)));



krondelta=abs(coe1(1:5)-coe(1:5))<=cutoff_coe(1:5);
controlling=activecorr_coe(1:5).*(1-krondelta);
controlling(1)=controlling(1) &  coe(2)<=.99;
controlling(5)=controlling(5) &  ~any(controlling(1:4));

dv_sma  = abs(V-V1);
dv_ecc  = V1*2/3*abs(asin(coe(2))-asin(coe1(2)));
dv_incl = V1*sqrt(2-2*cos(pi/2*(coe1(3)-coe(3))));
dv_an   = V1*pi/2*abs(coe1(4)-coe(4))*sin(coe1(3));
dv_ap   = V1*2/3*coe1(2)/sqrt(1-coe1(2)^2)*abs(coe1(5)-coe(5));

% a=zeros(5,1);
% b=zeros(5,1);
% eff=zeros(5,1);



a=zeros(5,1);
b=zeros(5,1);
eff=zeros(5,1);
tranmax=zeros(5,1);

T=zeros(5,3);
%SMA
ii=1;
a(ii)=atan(ecc*sin(tran)/(1+ecc*cos(eccan)));
b(ii)=0;
tranmax(ii)=0;
r=sma*(1-ecc^2)/(1+ecc*cos(tran));
rp=sma*(1-ecc^2)/(1+ecc*cos(tranmax(ii)));
%eff(ii)=(sqrt(sma*(2/r-1/sma)*(1-ecc)/(1+ecc)))/...
%    (sqrt(sma*(2/rp-1/sma)*(1-ecc)/(1+ecc)));
eff(ii)=sqrt(mu*(2/r-1/sma))*sqrt(sma*(1-ecc))/sqrt(mu*(1+ecc));

(sqrt(sma*(2/r-1/sma)*(1-ecc)/(1+ecc)))/...
    (sqrt(sma*(2/rp-1/sma)*(1-ecc)/(1+ecc)));

[c,r,nn]= sph2cart(a(ii),-b(ii),1);
T(ii,1)=c;
T(ii,2)=nn;
T(ii,3)=-r;

T(ii,:)=T(ii,:)*sign((coe1(ii)-coe(ii)));

%ECC
ii=2;
a(ii)=atan2(sin(tran),(cos(tran)+cos(eccan)));
b(ii)=0;
tranmax(ii)=pi;
%eff(ii)=(2*(1+2*ecc*cos(tran)+cos(tran)^2)/(1+ecc*cos(tran)))/...
%    (2*(1+2*ecc*cos(tranmax(ii))+cos(tranmax(ii))^2)/(1+ecc*cos(tranmax(ii))));
eff(ii)=(1/2*(1+2*ecc*cos(tran)+cos(tran)^2)/(1+ecc*cos(tran)));
[c,r,nn]= sph2cart(a(ii),-b(ii),1);
T(ii,1)=c;
T(ii,2)=nn;
T(ii,3)=-r;
T(ii,:)=T(ii,:)*sign((coe1(ii)-coe(ii)));%*sign(cos(tran));

%Incl
ii=3;
a(ii)=0;
b(ii)=sign(cos(ap+tran))*pi/2;
tranmax(ii)=asin(-ecc*sin(ap))-ap;
eff(ii)=(abs(cos(ap+tran))/(1+ecc*cos(tran)) *(sqrt(1-ecc^2*sin(ap)^2)-ecc*abs(cos(ap))));
[c,r,nn]= sph2cart(a(ii),-b(ii),1);
T(ii,1)=c;
T(ii,2)=nn;
T(ii,3)=-r;
T(ii,:)=T(ii,:)*sign((coe1(ii)-coe(ii)));

%RAAN
ii=4;
a(ii)=0;
b(ii)=sign(sin(ap+tran))*pi/2;
tranmax(ii)=acos(-ecc*cos(ap))-ap;
eff(ii)=(abs(sin(ap+tran))/(1+ecc*sin(tran))*(sqrt(1-ecc^2*cos(ap)^2)-ecc*abs(sin(ap))));
[c,r,nn]= sph2cart(a(ii),-b(ii),1);
T(ii,1)=c;
T(ii,2)=nn;
T(ii,3)=-r;
T(ii,:)=T(ii,:)*sign((coe1(ii)-coe(ii)));

%AP %WARNING! the AP control law does not appear to be correct.
ii=5;
if ecc>0
    if 0
        a(ii) = tran - pi/2;
        b(ii) = 0;
        
        
    else
        
        
        a(ii) = atan((1+ecc*cos(tran))/(2+ecc*cos(tran))*cot(tran));
        b(ii) = atan((ecc*cot(incl)*sin(ap+tran))/(sin(a(ii)-tran)*(1+ecc*cos(tran))-cos(a(ii))*sin(tran)));
        u     = (1-ecc^2)/ecc^3;
        v     = sqrt(1/4*u^2+1/27);
        costranmax=sign(u+v)*(abs(u+v))^(1/3)-sign((-u+v))*(abs(-u+v))^(1/3)-1/ecc;
        if costranmax>1
            costranmax=1;
        elseif costranmax<-1
            costranmax=-1;
        end
        tranmax(ii)=acos(costranmax);
        eff(ii)=((1+sin(tran)^2)/(1+ecc*cos(tran))*(1+ecc*cos(tranmax(ii)))/(1+sin(tranmax(ii))^2));
    end
else
    a(ii)=0;
    b(ii)=0;
    eff(ii)=0;
end
[c,r,nn]= sph2cart(a(ii),-b(ii),1);
T(ii,1)=c;
T(ii,2)=nn;
T(ii,3)=-r;
T(ii,:)=T(ii,:)*sign((coe1(ii)-coe(ii)));





%Waithted by ratio
denom=(coe1(1:5)-coe0(1:5));
temp=cutoff_coe(1:5);
denom(abs(denom) <=temp)=temp(abs(denom) <=temp)*10;
%denom(4)=denom(3);
weights=(coe1(1:5)-coe(1:5))./denom.*activecorr_coe(1:5).*balanced_coe;

weights(denom==0)=1;
weights=abs(weights);

%Weighted by ratio of dv
%weights=[dv_sma dv_ecc, dv_incl, dv_an, dv_ap]'.*activecorr_coe(1:5);
weights=reshape(weights,5,1).*controlling;
weights(isnan(weights))=0;
magn=sum(abs(weights));
if magn>0
    weights=weights/magn;
else
    weights=weights*0;
end

% krondelta(2)=krondelta(2) |  (coe(1)-coe0(1))/(coe1(1)-coe0(1))<.5;
% krondelta(3)=krondelta(3) ;

temp=activecorr_coe(1:5).*controlling.*eff.*weights;
magn=sum(abs(temp));
if magn>0
    temp=temp/magn;
else
    temp=temp*0;
end

Ttemp=sum(temp'*T,1);
nT_slo=Ttemp/norm(Ttemp);
nT_slo(isnan(nT_slo))=0;


[alpha,beta]=cart2sph(nT_slo(:,1),-nT_slo(:,2),-nT_slo(:,3));
alpha=-alpha;

== matlab function HSat_orbit_merged_maria/Subsystem1/Navigation/Subsystem/Subsystem/MATLAB Function ==
  data: r input; coe output; v input
%SV2KEP.M
%
%function kepvec=sv2kep(rsc,vsc)
%
%DESCRIPTION
%Converts from state vector (rvec,vvec) formulation to keplerian elements
%
%INPUT:		rsc	 (3x1) or (3xn) orbit radius vector
%				vsc (3x1) or (3xn) velocity vector
%
%OUTPUT:    	kepvec - (6x1) or (6xn) vector with the keplerian elements
%USES:
%REFERENCE:
%AUTHOR:      	B Jakobsson
%VERSION: 	   92-08-17
%	   	      95-10-02
%				BJA, Sept 2001, vector input accepted, vector output added

% function coe=sv2kep(rvec,vvec)
% 
% if 0
% [p,sma,ecc,incl,an,ap,tran,E,M,arglat,truelon,lonper ] = rv2coe (rvec,vvec);
% coe=[sma ecc incl an ap tran, E, M,arglat,truelon,lonper ]';
% else
%     coe = rv2coe (rvec,vvec);
% end
  
%
% ------------------------------------------------------------------------------
%
%                           function rv2coe
%
%  this function finds the classical orbital elements given the geocentric
%    equatorial position and velocity vectors.
%
%  author        : david vallado                  719-573-2600   21 jun 2002
%
%  revisions
%    vallado     - fix special cases                              5 sep 2002
%    vallado     - delete extra check in inclination code        16 oct 2002
%    vallado     - add constant file use                         29 jun 2003
%    vallado     - add mu                                         2 apr 2007
%
%  inputs          description                    range / units
%    r           - ijk position vector            km
%    v           - ijk velocity vector            km / s
%    mu          - gravitational parameter        km3 / s2
%
%  outputs       :
%    p           - semilatus rectum               km
%    a           - semimajor axis                 km
%    ecc         - eccentricity
%    incl        - inclination                    0.0  to pi rad
%    omega       - longitude of ascending node    0.0  to 2pi rad
%    argp        - argument of perigee            0.0  to 2pi rad
%    nu          - true anomaly                   0.0  to 2pi rad
%    m           - mean anomaly                   0.0  to 2pi rad
%    arglat      - argument of latitude      (ci) 0.0  to 2pi rad
%    truelon     - true longitude            (ce) 0.0  to 2pi rad
%    lonper      - longitude of periapsis    (ee) 0.0  to 2pi rad
%
%  locals        :
%    hbar        - angular momentum h vector      km2 / s
%    ebar        - eccentricity     e vector
%    nbar        - line of nodes    n vector
%    c1          - v**2 - u/r
%    rdotv       - r dot v
%    hk          - hk unit vector
%    sme         - specfic mechanical energy      km2 / s2
%    i           - index
%    e           - eccentric, parabolic,
%                  hyperbolic anomaly             rad
%    temp        - temporary variable
%    typeorbit   - type of orbit                  ee, ei, ce, ci
%
%  coupling      :
%    mag         - magnitude of a vector
%    angl        - find the angl between two vectors
%    newtonnu    - find the mean anomaly
%
%  references    :
%    vallado       2007, 121, alg 9, ex 2-5
%
% [p,a,ecc,incl,omega,argp,nu,m,arglat,truelon,lonper ] = rv2coe (r,v);
% ------------------------------------------------------------------------------

  %  function [p,a,ecc,incl,omega,argp,nu,e,m,arglat,truelon,lonper ] = rv2coe (r,v);
     function coe = rv2coe (r,v)
        
        %  constmath;
        small=1e-10;
        infinite  = 999999.9;
        undefined = 999999.1;
        % -------------------------  mathematical  --------------------
        rad    = 180.0 / pi;
        twopi  = 2.0 * pi;
        halfpi = pi * 0.5;
        
        % constastro;  % don't overwrite mu
        mu=3.986005e14;
        muin = mu; % this is the km version
        % -------------------------  implementation   -----------------
        magr = norm( r );
        magv = norm( v );
        % ------------------  find h n and e vectors   ----------------
        [hbar] = cross( r,v );
        nbar=hbar*NaN;
        ebar=hbar*NaN;
        magh = mag( hbar );
        if ( magh > small )
            nbar(1)= -hbar(2);
            nbar(2)=  hbar(1);
            nbar(3)=   0.0;
            magn = mag( nbar );
            c1 = magv*magv - muin /magr;
            rdotv= dot( r,v );
            for i= 1 : 3
                ebar(i)= (c1*r(i) - rdotv*v(i))/muin;
            end
            ecc = mag( ebar );
            
            % ------------  find a e and semi-latus rectum   ----------
            sme= ( magv*magv*0.5  ) - ( muin /magr );
            if ( abs( sme ) > small )
                a= -muin  / (2.0 *sme);
            else
                a= infinite;
            end
            p = magh*magh/muin;
            
            % -----------------  find inclination   -------------------
            hk= hbar(3)/magh;
            incl= acos( hk );
            
            % --------  determine type of orbit for later use  --------
            % ------ elliptical, parabolic, hyperbolic inclined -------
            typeorbit= 'ei';
            if ( ecc < small )
                % ----------------  circular equatorial ---------------
                if  (incl<small) || (abs(incl-pi)<small)
                    typeorbit= 'ce';
                else
                    % --------------  circular inclined ---------------
                    typeorbit= 'ci';
                end
            else
                % - elliptical, parabolic, hyperbolic equatorial --
                if  (incl<small) || (abs(incl-pi)<small)
                    typeorbit= 'ee';
                end
            end
            
            % ----------  find longitude of ascending node ------------
            if ( magn > small )
                temp= nbar(1) / magn;
                if ( abs(temp) > 1.0  )
                    temp= sign(temp);
                end
                omega= acos( temp );
                if ( nbar(2) < 0.0  )
                    omega= twopi - omega;
                end
            else
                omega= undefined;
            end
            
            % ---------------- find argument of perigee ---------------
            if (strcmp(typeorbit, 'ei') == 1)
                argp = angl( nbar,ebar);
                if ( ebar(3) < 0.0  )
                    argp= twopi - argp;
                end
            else
                argp= undefined;
            end
            
            % ------------  find true anomaly at epoch    -------------
            if ( typeorbit(1:1) == 'e' )
                nu =  angl( ebar,r);
                if ( rdotv < 0.0  )
                    nu= twopi - nu;
                end
            else
                nu= undefined;
            end
            
            % ----  find argument of latitude - circular inclined -----
            if (strcmp(typeorbit, 'ci') == 1)
                arglat = angl( nbar,r );
                if ( r(3) < 0.0  )
                    arglat= twopi - arglat;
                end
                m = arglat;
            else
                arglat= undefined;
            end
            
            % -- find longitude of perigee - elliptical equatorial ----
            if  ( ecc>small ) && (strcmp(typeorbit, 'ee') == 1)
                temp= ebar(1)/ecc;
                if ( abs(temp) > 1.0  )
                    temp= sign(temp);
                end
                lonper= acos( temp );
                if ( ebar(2) < 0.0  )
                    lonper= twopi - lonper;
                end
                if ( incl > halfpi )
                    lonper= twopi - lonper;
                end
            else
                lonper= undefined;
            end
            
            % -------- find true longitude - circular equatorial ------
            if  ( magr>small ) && (strcmp(typeorbit, 'ce') == 1)
                temp= r(1)/magr;
                if ( abs(temp) > 1.0  )
                    temp= sign(temp);
                end
                truelon= acos( temp );
                if ( r(2) < 0.0  )
                    truelon= twopi - truelon;
                end
                if ( incl > halfpi )
                    truelon= twopi - truelon;
                end
                m = truelon;
            else
                truelon= undefined;
            end
            
            % ------------ find mean anomaly for all orbits -----------
            if ( typeorbit(1:1) == 'e' )
                [e,m] = newtonnu(ecc,nu );
                e=mod(e,2*pi);
            else
                e=undefined;
                m=undefined;
                
            end
            
        else
            p    = undefined;
            a    = undefined;
            ecc  = undefined;
            incl = undefined;
            omega= undefined;
            argp = undefined;
            nu   = undefined;
            m    = undefined;
            e    = undefined;
            arglat = undefined;
            truelon= undefined;
            lonper = undefined;
        end
%coe=[sma ecc incl an ap tran, E, M,arglat,truelon,lonper ]
coe=[  a,ecc,incl,omega,argp,nu,e,m,arglat,truelon,lonper ]';
    end
% end

== matlab function HSat_orbit_merged_maria/Subsystem1/control/TorquesAndForces/MATLAB Function ==
  data: v input; u output; w input
function u = cross(v,w)

u = cross(v,w,2);

== matlab function HSat_orbit_merged_maria/Subsystem1/Dynamics/Subsystem/3 body perturbation legendre polynomial/Subsystem1/MATLAB Function ==
  data: costheta input; beta output; degree input; h input
function beta = beta_f(costheta, degree, h)
B = -1;
P = zeros(1, degree+1);
for d = 0:degree
    if d == 0
        P(d+1) = 1;
    elseif d == 1
            P(d+1) = costheta;
    else
        P(d+1) = (2*d-1)/d*costheta*P(d)-(d-1)/d*P(d-1);
    end
    B = B + P(d+1)*h^d;
end
beta = 3*B + 3*B^2 + B^3;

== matlab function HSat_orbit_merged_maria/Subsystem1/Dynamics/Subsystem/3 body perturbation legendre polynomial/Subsystem2/MATLAB Function ==
  data: costheta input; beta output; degree input; h input
function beta = beta_f(costheta, degree, h)
B = -1;
P = zeros(1, degree+1);
for d = 0:degree
    if d == 0
        P(d+1) = 1;
    elseif d == 1
            P(d+1) = costheta;
    else
        P(d+1) = (2*d-1)/d*costheta*P(d)-(d-1)/d*P(d-1);
    end
    B = B + P(d+1)*h^d;
end
beta = 3*B + 3*B^2 + B^3;

== matlab function HSat_orbit_merged_maria/Subsystem1/Dynamics/Subsystem/3 body perturbation legendre polynomial/Subsystem3/MATLAB Function ==
  data: costheta input; beta output; degree input; h input
function beta = beta_f(costheta, degree, h)
B = -1;
P = zeros(1, degree+1);
for d = 0:degree
    if d == 0
        P(d+1) = 1;
    elseif d == 1
            P(d+1) = costheta;
    else
        P(d+1) = (2*d-1)/d*costheta*P(d)-(d-1)/d*P(d-1);
    end
    B = B + P(d+1)*h^d;
end
beta = 3*B + 3*B^2 + B^3;
